simulink model "lqr_pendubot"  (R2021a)
settings: Solver=ode4  StartTime=0.0  StopTime=20  FixedStep=0.01  RelTol=1e-3
values from neighbouring files (symbols this model uses):
  COEFF = [a1 a2 a3 a4 a5 f1 f2]    [lqr_init.m]
  INITIAL_CONDITIONS = [0,0,0,0]    [Alternative_Init.m]    (also in init.m = [-pi/2,0,0,0]; lqr_init.m = [pi + pi/12, -pi/12, 0, 0])
  K_d = -K(3:4)    [DaCBarF.m]    (also in Pendubot_init.m; Segway_paper.m = 0.1; lqr_init.m)
  K_p = -K(1:2)    [DaCBarF.m]    (also in Pendubot_init.m; Segway_paper.m = 1; lqr_init.m)
  lb = -100    [lqr_init.m]
  q1e = pi    (= 3.14159265359)    [Pendubot_init.m]    (also in lqr_init.m = 2.87979326579)
  q2e = pi - Q1E    (= 0)    [Pendubot_init.m]    (also in lqr_init.m = 0.261799387799)
  Q_DES = [X_EQ; THETA_EQ]    [Cartpole.m]    (also in DaCBarF.m = [Q1E; Q2E]; Pendubot_init.m = [q1e; q2e]; lqr_init.m = [q1e; q2e])
  tau_eq = mp*G*l*sin(thetae)    [Cartpole.m]    (also in DaCBarF.m = a4*sin(Q1E)+a5*sin(Q1E+Q2E); Pendubot_init.m = [a4*sin(q1e)+a5*sin(q1e+q2e)]; lqr_init.m = [a4*sin(q1e)+a5*sin(q1e+q2e)])
  ub = 100    [lqr_init.m]
settings Model: Creator=lorenzo  LastModifiedBy=gianl
settings SolverCC: AlgebraicLoopSolver=TrustRegion
settings DataIOCC: InspectSignalLogs=on  ReturnWorkspaceOutputs=off
settings DebuggingCC: SFMachineParentedDataDiag=warning

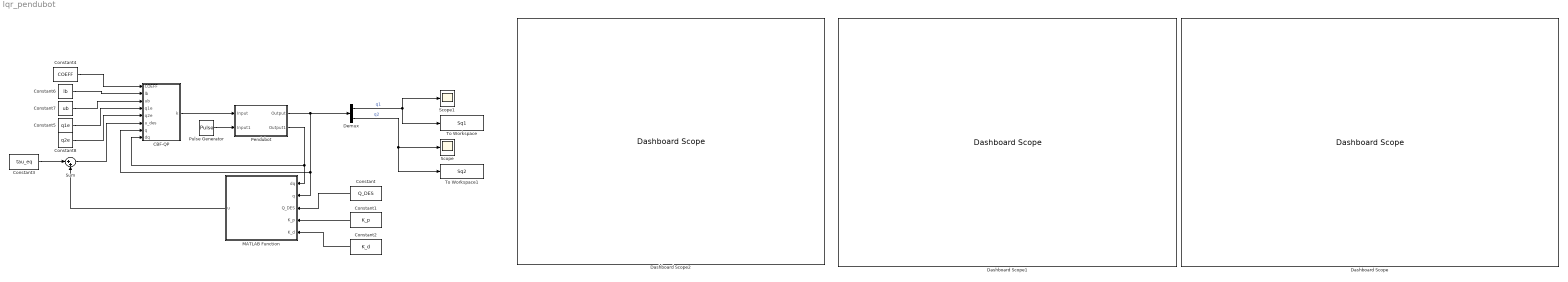
== system lqr_pendubot ==
  CBF-QP : MATLAB Function  TreatAsAtomicUnit=on
  Constant : Constant  Value=Q_DES
  Constant1 : Constant  Value=K_p
  Constant2 : Constant  Value=K_d
  Constant3 : Constant  Value=tau_eq
  Constant4 : Constant  Value=COEFF
  Constant5 : Constant  Value=q1e
  Constant6 : Constant  Value=lb
  Constant7 : Constant  Value=ub
  Constant8 : Constant  Value=q2e
  Dashboard Scope : DashboardScope
  Dashboard Scope1 : DashboardScope
  Dashboard Scope2 : DashboardScope
  Demux : Demux  Outputs=2
  MATLAB Function : MATLAB Function  TreatAsAtomicUnit=on
  Pendubot : Subsystem
  Pulse Generator : DiscretePulseGenerator  PulseType=Time based  Period=10
  Scope : Scope
  Scope1 : Scope
  Sum : Sum  Inputs=|++
  To Workspace : ToWorkspace  VariableName=Sq1  SaveFormat=Timeseries  SampleTime=-1
  To Workspace1 : ToWorkspace  VariableName=Sq2  SaveFormat=Timeseries  SampleTime=-1
  wires:
  Pendubot/1(Output) -> Demux/1, CBF-QP/7(q), MATLAB Function/2(q)
  Pendubot/2(Output1) -> MATLAB Function/1(dq), CBF-QP/8(dq)
  Constant/1 -> MATLAB Function/3(Q_DES)
  Constant1/1 -> MATLAB Function/4(K_p)
  Constant2/1 -> MATLAB Function/5(K_d)
  MATLAB Function/1(u) -> Sum/2
  Constant3/1 -> Sum/1
  Demux/1 -> Scope1/1, To Workspace/1  "q1"
  Demux/2 -> To Workspace1/1, Scope/1  "q2"
  CBF-QP/1(k) -> Pendubot/1(Input)
  Sum/1 -> CBF-QP/6(u_des)
  Constant6/1 -> CBF-QP/2(lb)
  Constant7/1 -> CBF-QP/3(ub)
  Constant8/1 -> CBF-QP/5(q2e)
  Constant4/1 -> CBF-QP/1(COEFF)
  Constant5/1 -> CBF-QP/4(q1e)
  Pulse Generator/1 -> Pendubot/2(Input1)

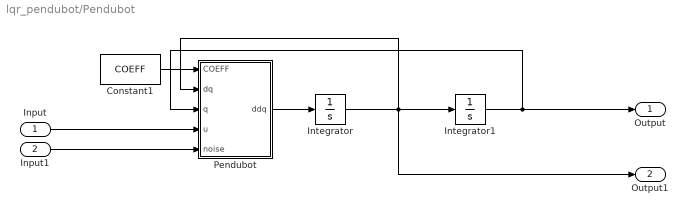
== system lqr_pendubot/Pendubot ==
  Input : Inport
  Input1 : Inport  Port=2
  Constant1 : Constant  Value=COEFF
  Integrator : Integrator  InitialCondition=INITIAL_CONDITIONS(3:4)
  Integrator1 : Integrator  InitialCondition=INITIAL_CONDITIONS(1:2)
  Pendubot : MATLAB Function  TreatAsAtomicUnit=on
  Output : Outport
  Output1 : Outport  Port=2
  wires:
  Pendubot/1(ddq) -> Integrator/1
  Integrator1/1 -> Output/1, Pendubot/3(q)
  Integrator/1 -> Output1/1, Pendubot/2(dq), Integrator1/1
  Input/1 -> Pendubot/4(u)
  Constant1/1 -> Pendubot/1(COEFF)
  Input1/1 -> Pendubot/5(noise)

== matlab function lqr_pendubot/MATLAB Function ==
  data: dq input size=[2 1]; u output size=1; q input size=[2 1]; Q_DES input size=[2 1]; K_p input size=[1 2]; K_d input size=[ 1 2]
function u = lqr_controller(dq,q,Q_DES,K_p,K_d)

tau = K_p*(q-Q_DES) + K_d*dq;

u = tau;

== matlab function lqr_pendubot/Pendubot/Pendubot ==
  data: COEFF input; dq input; q input; u input; ddq output; noise input
function ddq = fcn(COEFF,dq,q,u,noise)

a1 = COEFF(1);
a2 = COEFF(2);
a3 = COEFF(3);
a4 = COEFF(4);
a5 = COEFF(5);

f1 = COEFF(6);
f2 = COEFF(7);

q1 = q(1);
q2 = q(2);
dq1 = dq(1);
dq2 = dq(2);

M = [a1 + 2*a2*cos(q2), a3+a2*cos(q2);
     a3+a2*cos(q2),          a3];

F = diag([f1,f2]);

e = [a4*sin(q1)+a5*sin(q1+q2);
            a5*sin(q1+q2)];

c = [a2*sin(q2)*dq2*(dq2+2*dq1);
         a2*sin(q2)*dq1^2];

ddq = M\(u-F*dq-c-e-noise);

== matlab function lqr_pendubot/CBF-QP ==
  data: COEFF input; lb input; ub input; q1e input; q2e input; u_des input size=1; q input; dq input; k output size=[2,1]
function k = cbfqp(COEFF, lb, ub, q1e, q2e, u_des, q, dq)

a1 = COEFF(1);
a2 = COEFF(2);
a3 = COEFF(3);
a4 = COEFF(4);
a5 = COEFF(5);

f1 = COEFF(6);
f2 = COEFF(7);

q1 = q(1);
q2 = q(2);
dq1 = dq(1);
dq2 = dq(2);

M = [a1 + 2*a2*cos(q2), a3+a2*cos(q2);
     a3+a2*cos(q2),          a3];

F = diag([f1,f2]);

e = [a4*sin(q1)+a5*sin(q1+q2);
            a5*sin(q1+q2)];

c = [a2*sin(q2)*dq2*(dq2+2*dq1);
         a2*sin(q2)*dq1^2];

f_sys = [dq1; dq2; M\(-F*dq-c-e)];
g_sys = [0 0; 0 0; inv(M)];


Q2E_MAX = pi/12;
c = 0.1;
alpha = 1;
cbf = 0.5*(Q2E_MAX^2-(q2-q2e)^2-c*dq2^2);
grad = [q1e - q1, 0, -c*dq1, 0];

Aeq = [];
beq = [];

H = eye(2);
f = -[u_des; 0];
A = -grad*g_sys;
b = grad*f_sys+alpha*cbf;

options = optimoptions('quadprog','Algorithm','active-set');

u_qp = quadprog(H,f,A,b,Aeq,beq,[],[],[u_des,0]',options);
%u_qp = [u_des,0]';

k = u_qp;
